simulink model "V.1.3.SystemsmModelling_Modified_Aircorn"  (R2020a)
settings: Solver=ode23t  StartTime=0.0  StopTime=2000  MaxStep=2000.0  RelTol=1e-3
values from neighbouring files (symbols this model uses):
  InitialTemp = 300    [Setup.m]
undefined symbols (not defined in the file or in its folder): commanded_mass_flow, compressor_time_constant, condenser_length, copper_density, environment_temperature, evaporator_length, ground_temperature, pipe_diameter, pipe_thickness, target_temperature, temperature_delta, u_sat
libraries: fl_lib x55, nesl_utility x8, refrigeration_lib x1
(part 3 of 3)

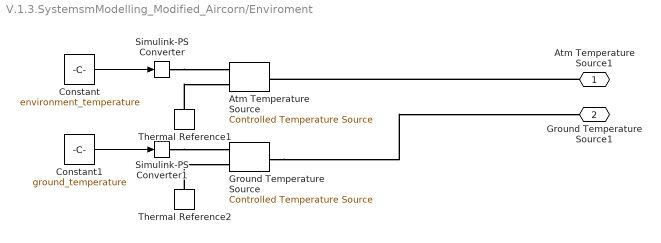
== system V.1.3.SystemsmModelling_Modified_Aircorn/Enviroment ==
  Atm Temperature Source : fl_lib/Thermal/Thermal Sources/Controlled Temperature Source
  Constant : Constant  Value=environment_temperature
  Constant1 : Constant  Value=ground_temperature
  Ground Temperature Source : fl_lib/Thermal/Thermal Sources/Controlled Temperature Source
  Simulink-PS Converter : nesl_utility/Simulink-PS Converter  PhysicalDomain=network_engine_domain  SubClassName=ps_input  LeftPortType=input  RightPortType=output  PseudoPeriodic=off  Frequencies=[]  NoiseDistribution=none  NoiseParameters=[]  Unit=1  AffineConversion=off  FilteringAndDerivatives=provide  SimscapeFilterOrder=1  InputFilterTimeConstant=0.001  UdotUserProvided=0
  Simulink-PS Converter1 : nesl_utility/Simulink-PS Converter  PhysicalDomain=network_engine_domain  SubClassName=ps_input  LeftPortType=input  RightPortType=output  PseudoPeriodic=off  Frequencies=[]  NoiseDistribution=none  NoiseParameters=[]  Unit=1  AffineConversion=off  FilteringAndDerivatives=provide  SimscapeFilterOrder=1  InputFilterTimeConstant=0.001  UdotUserProvided=0
  Thermal Reference1 : fl_lib/Thermal/Thermal Elements/Thermal Reference
  Thermal Reference2 : fl_lib/Thermal/Thermal Elements/Thermal Reference
  Atm Temperature Source1 : PMIOPort  Side=Left
  Ground Temperature Source1 : PMIOPort  Port=2  Side=Left
  wires:
  Constant/1 -> Simulink-PS Converter/1
  Constant1/1 -> Simulink-PS Converter1/1
  connections:
  Thermal Reference2/LConn1 -- Ground Temperature Source/RConn2
  Thermal Reference1/LConn1 -- Atm Temperature Source/RConn2
  Simulink-PS Converter1/RConn1 -- Ground Temperature Source/RConn1
  Ground Temperature Source/LConn1 -- Ground Temperature Source1/RConn1
  Atm Temperature Source1/RConn1 -- Atm Temperature Source/LConn1
  Simulink-PS Converter/RConn1 -- Atm Temperature Source/RConn1

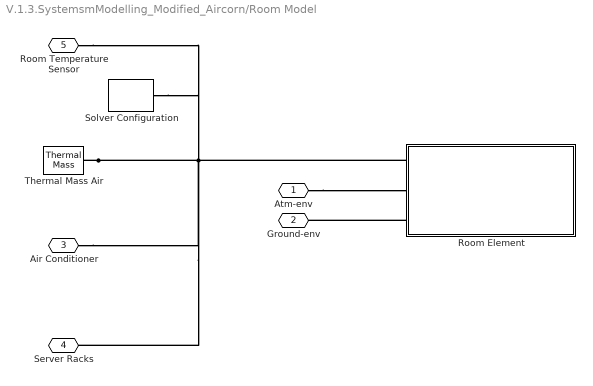
== system V.1.3.SystemsmModelling_Modified_Aircorn/Room Model ==
  "Room Element " : Subsystem
  Solver Configuration : nesl_utility/Solver Configuration  PhysicalDomain=network_engine_domain  SubClassName=solver  LeftPortType=input  RightPortType=generic  Tones=[]  Harmonics=[]  SimulateNoise=off  Profile=off  UseLocalSampling=off  EnableSwitchedLinearOptims=on  FrequencyDomain=off  UseCCode=off  RelTol=0.001  AbsTol=1e-06  MinStep=1e-09  ToWorkspace=off  RevertToSquareIcSolve=off  NumHomotopyIterations=100  PhasorMode=off  PhasorModeNumHarmonics=1  DoDC=off  ResidualTolerance=1e-09  UseLocalSolver=off  LocalSolverChoice=NE_BACKWARD_EULER_ADVANCER  LocalSolverSampleTime=0.001  DoFixedCost=off  MaxNonlinIter=3  MaxModeIter=2  LinearAlgebra=auto  EquationFormulation=NE_TIME_EF  DelaysMemoryBudget=1024  AutomaticFiltering=on  FilteringTimeConstant=0.001  PartitionStorageMethod=AS_NEEDED  PartitionMemoryBudget=1024  PartitionMethod=ROBUST
  Thermal Mass Air : fl_lib/Thermal/Thermal Elements/Thermal Mass  mass=1 kg  sp_heat=1012 J/kg/K  T_specify=off  T_priority=High  T=300 K  T_nominal_specify=off  T_nominal_unit=K  T_nominal_value=1  Q_specify=off  Q_priority=None  Q=0 W  Q_nominal_specify=off  Q_nominal_unit=W  Q_nominal_value=1
  Atm-env : PMIOPort  Side=Left
  Ground-env : PMIOPort  Port=2  Side=Left
  Air Conditioner : PMIOPort  Port=3  Side=Left
  Server Racks : PMIOPort  Port=4  Side=Left
  "Room Temperature Sensor " : PMIOPort  Port=5  Side=Left
  connections:
  Thermal Mass Air/LConn1 -- Server Racks/RConn1 -- Air Conditioner/RConn1 -- "Room Temperature Sensor "/RConn1 -- Solver Configuration/RConn1 -- "Room Element "/LConn1
  Atm-env/RConn1 -- "Room Element "/LConn2
  "Room Element "/LConn3 -- Ground-env/RConn1

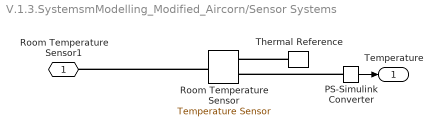
== system V.1.3.SystemsmModelling_Modified_Aircorn/Sensor Systems ==
  PS-Simulink Converter : nesl_utility/PS-Simulink Converter  PhysicalDomain=network_engine_domain  SubClassName=ps_output  LeftPortType=input  RightPortType=output  PseudoPeriodic=off  Frequencies=[]  Unit=inherit  AffineConversion=off
  Room Temperature Sensor : fl_lib/Thermal/Thermal Sensors/Temperature Sensor
  Thermal Reference : fl_lib/Thermal/Thermal Elements/Thermal Reference
  Room Temperature Sensor1 : PMIOPort  Side=Left
  "Temperature " : Outport
  wires:
  PS-Simulink Converter/1 -> "Temperature "/1
  connections:
  PS-Simulink Converter/LConn1 -- Room Temperature Sensor/RConn2
  Thermal Reference/LConn1 -- Room Temperature Sensor/RConn1
  Room Temperature Sensor/LConn1 -- Room Temperature Sensor1/RConn1

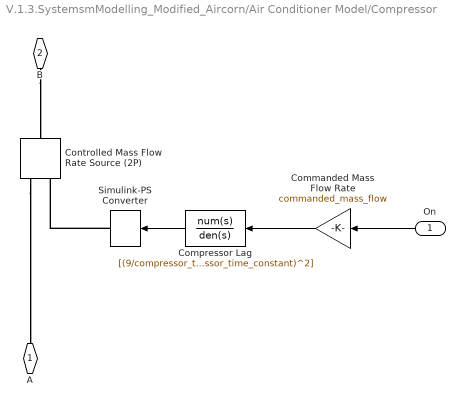
== system V.1.3.SystemsmModelling_Modified_Aircorn/Air Conditioner Model/Compressor ==
  On : Inport
  Commanded Mass Flow Rate : Gain  Gain=commanded_mass_flow
  Compressor Lag : TransferFcn  Numerator=[(9/compressor_time_constant)^2]  Denominator=[1, 2*(9/compressor_time_constant), (9/compressor_time_constant)^2]
  Controlled Mass Flow Rate Source (2P) : fl_lib/Two-Phase Fluid/Sources/Controlled Mass Flow Rate Source (2P)  power_spec=foundation.enum.power_spec.isentropic  area_A=pi*pipe_diameter^2/4 m^2  area_B=pi*pipe_diameter^2/4 m^2
      settings: SourceProductBaseCode=SS  InternalSimscapePortConfiguration="{\"Bottom\":[],\"Left\":[{\"id\":\"A\",\"label\":\"A\",\"type\":\"foundation.two_phase_fluid.two_phase_fluid\"},{\"id\":\"M\",\"label\":\"M\",\"type\":\"input\"}],\"Right\":[{\"id\":\"B\",\"label\":\"B\",\"type\":\"foundation.two_phase_fluid.two_phase_fluid\"}],\"Top\":[]}"
  Simulink-PS Converter : nesl_utility/Simulink-PS Converter  PhysicalDomain=network_engine_domain  SubClassName=ps_input  LeftPortType=input  RightPortType=output  PseudoPeriodic=off  Frequencies=[]  NoiseDistribution=none  NoiseParameters=[]  Unit=kg/s  AffineConversion=off  FilteringAndDerivatives=zero  SimscapeFilterOrder=1  InputFilterTimeConstant=0.001  UdotUserProvided=1
  A : PMIOPort  Side=Left
  B : PMIOPort  Port=2  Side=Right
  wires:
  Compressor Lag/1 -> Simulink-PS Converter/1
  Commanded Mass Flow Rate/1 -> Compressor Lag/1
  On/1 -> Commanded Mass Flow Rate/1
  connections:
  Simulink-PS Converter/RConn1 -- Controlled Mass Flow Rate Source (2P)/LConn2
  Controlled Mass Flow Rate Source (2P)/LConn1 -- A/RConn1
  B/RConn1 -- Controlled Mass Flow Rate Source (2P)/RConn1

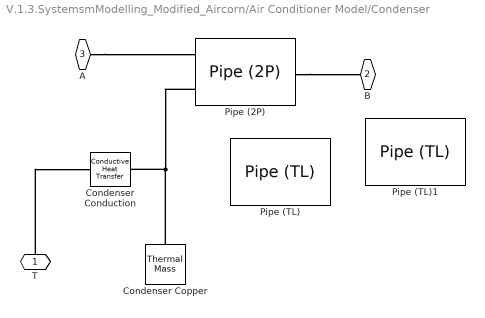
== system V.1.3.SystemsmModelling_Modified_Aircorn/Air Conditioner Model/Condenser ==
  Condenser Conduction : fl_lib/Thermal/Thermal Elements/Conductive Heat Transfer  area=pi*pipe_diameter*condenser_length m^2  thickness=pipe_thickness m  th_cond=copper_conductivity W/(m*K)  T_specify=off  T_priority=High  T=0 K  T_nominal_specify=off  T_nominal_unit=K  T_nominal_value=1  Q_specify=off  Q_priority=High  Q=0 J/s  Q_nominal_specify=off  Q_nominal_unit=W  Q_nominal_value=1
  Condenser Copper : fl_lib/Thermal/Thermal Elements/Thermal Mass  mass=pi*pipe_diameter*condenser_length*pipe_thickness*copper_density kg  sp_heat=copper_specific_heat J/kg/K  T_specify=on  T_priority=High  T=environment_temperature K  T_nominal_specify=off  T_nominal_unit=K  T_nominal_value=1  Q_specify=off  Q_priority=High  Q=0 J/s  Q_nominal_specify=off  Q_nominal_unit=W  Q_nominal_value=1
  Pipe (2P) : fl_lib/Two-Phase Fluid/Elements/Pipe (2P)  length=condenser_length m  area=pi*pipe_diameter^2/4 m^2  Dh=pipe_diameter m  length_add=0.1*condenser_length m  roughness=15e-6 m  Re_lam=2000  Re_tur=4000  shape_factor=64  Nu_lam=5  inertia=simscape.enum.onoff.off  energy_spec=foundation.enum.energy_spec.temperature  p_init=charge_pressure MPa  T_init=-1 K  x_init=0.5  alpha_init=0.5  h_init=1500 kJ/kg  u_init=1500 kJ/kg  mdot_init=0 kg/s  time_constant=0.1 s
      settings: SourceProductBaseCode=SS  InternalSimscapePortConfiguration="{\"Bottom\":[],\"Left\":[{\"id\":\"A\",\"label\":\"A\",\"type\":\"foundation.two_phase_fluid.two_phase_fluid\"},{\"id\":\"H\",\"label\":\"H\",\"type\":\"foundation.thermal.thermal\"}],\"Right\":[{\"id\":\"B\",\"label\":\"B\",\"type\":\"foundation.two_phase_fluid.two_phase_fluid\"}],\"Top\":[]}"
  Pipe (TL) : fl_lib/Thermal Liquid/Elements/Pipe (TL)  length=5 m  area=0.01 m^2  Dh=0.1128 m  length_add=1 m  roughness=15e-6 m  Re_lam=2000  Re_tur=4000  shape_factor=64  Nu_lam=3.66  dynamic_compressibility=simscape.enum.onoff.on  inertia=simscape.enum.onoff.off  p0=0.101325 MPa  T0=293.15 K  mdot0=0 kg/s
      settings: SourceProductBaseCode=SS
  Pipe (TL)1 : fl_lib/Thermal Liquid/Elements/Pipe (TL)  length=5 m  area=0.01 m^2  Dh=0.1128 m  length_add=1 m  roughness=15e-6 m  Re_lam=2000  Re_tur=4000  shape_factor=64  Nu_lam=3.66  dynamic_compressibility=simscape.enum.onoff.on  inertia=simscape.enum.onoff.off  p0=0.101325 MPa  T0=293.15 K  mdot0=0 kg/s
      settings: SourceProductBaseCode=SS
  T : PMIOPort  Side=Left
  B : PMIOPort  Port=2  Side=Left
  A : PMIOPort  Port=3  Side=Right
  connections:
  Condenser Copper/LConn1 -- Pipe (2P)/LConn2 -- Condenser Conduction/LConn1
  T/RConn1 -- Condenser Conduction/RConn1
  A/RConn1 -- Pipe (2P)/LConn1
  Pipe (2P)/RConn1 -- B/RConn1

== system V.1.3.SystemsmModelling_Modified_Aircorn/Air Conditioner Model/Control ==
  Err : Inport
  Relay : Relay  OnSwitchValue=temperature_delta  OffSwitchValue=-temperature_delta
  On : Outport
  wires:
  Err/1 -> Relay/1
  Relay/1 -> On/1

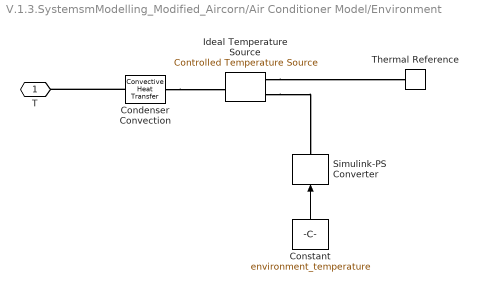
== system V.1.3.SystemsmModelling_Modified_Aircorn/Air Conditioner Model/Environment ==
  Condenser Convection : fl_lib/Thermal/Thermal Elements/Convective Heat Transfer  area=fin_area m^2  heat_tr_coeff=fin_convection_coefficient W/(m^2 * K)  T_specify=off  T_priority=High  T=0 K  T_nominal_specify=off  T_nominal_unit=K  T_nominal_value=1  Q_specify=off  Q_priority=High  Q=0 J/s  Q_nominal_specify=off  Q_nominal_unit=W  Q_nominal_value=1
  Constant : Constant  Value=environment_temperature
  Ideal Temperature Source : fl_lib/Thermal/Thermal Sources/Controlled Temperature Source
  Simulink-PS Converter : nesl_utility/Simulink-PS Converter  PhysicalDomain=network_engine_domain  SubClassName=ps_input  LeftPortType=input  RightPortType=output  PseudoPeriodic=off  Frequencies=[]  NoiseDistribution=none  NoiseParameters=[]  Unit=K  AffineConversion=off  FilteringAndDerivatives=zero  SimscapeFilterOrder=1  InputFilterTimeConstant=0.001  UdotUserProvided=1
  Thermal Reference : fl_lib/Thermal/Thermal Elements/Thermal Reference
  T : PMIOPort  Side=Left
  wires:
  Constant/1 -> Simulink-PS Converter/1
  connections:
  Condenser Convection/RConn1 -- Ideal Temperature Source/LConn1
  Condenser Convection/LConn1 -- T/RConn1
  Ideal Temperature Source/RConn1 -- Simulink-PS Converter/RConn1
  Ideal Temperature Source/RConn2 -- Thermal Reference/LConn1

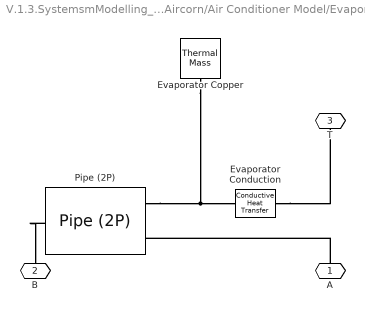
== system V.1.3.SystemsmModelling_Modified_Aircorn/Air Conditioner Model/Evaporator ==
  Evaporator Conduction : fl_lib/Thermal/Thermal Elements/Conductive Heat Transfer  area=pi*pipe_diameter*evaporator_length m^2  thickness=pipe_thickness m  th_cond=copper_conductivity W/(m*K)  T_specify=off  T_priority=High  T=0 K  T_nominal_specify=off  T_nominal_unit=K  T_nominal_value=1  Q_specify=off  Q_priority=High  Q=0 J/s  Q_nominal_specify=off  Q_nominal_unit=W  Q_nominal_value=1
  Evaporator Copper : fl_lib/Thermal/Thermal Elements/Thermal Mass  mass=pi*pipe_diameter*evaporator_length*pipe_thickness*copper_density kg  sp_heat=copper_specific_heat J/kg/K  T_specify=on  T_priority=High  T=target_temperature K  T_nominal_specify=off  T_nominal_unit=K  T_nominal_value=1  Q_specify=off  Q_priority=High  Q=0 J/s  Q_nominal_specify=off  Q_nominal_unit=W  Q_nominal_value=1
  Pipe (2P) : fl_lib/Two-Phase Fluid/Elements/Pipe (2P)  length=evaporator_length m  area=pi*pipe_diameter^2/4 m^2  Dh=pipe_diameter m  length_add=0.1*evaporator_length m  roughness=15e-6 m  Re_lam=2000  Re_tur=4000  shape_factor=64  Nu_lam=5  inertia=simscape.enum.onoff.off  energy_spec=foundation.enum.energy_spec.temperature  p_init=charge_pressure MPa  T_init=-1 K  x_init=0.5  alpha_init=0.5  h_init=1500 kJ/kg  u_init=1500 kJ/kg  mdot_init=0 kg/s  time_constant=0.1 s
      settings: SourceProductBaseCode=SS  InternalSimscapePortConfiguration="{\"Bottom\":[],\"Left\":[{\"id\":\"A\",\"label\":\"A\",\"type\":\"foundation.two_phase_fluid.two_phase_fluid\"},{\"id\":\"H\",\"label\":\"H\",\"type\":\"foundation.thermal.thermal\"}],\"Right\":[{\"id\":\"B\",\"label\":\"B\",\"type\":\"foundation.two_phase_fluid.two_phase_fluid\"}],\"Top\":[]}"
  A : PMIOPort  Side=Left
  B : PMIOPort  Port=2  Side=Right
  T : PMIOPort  Port=3  Side=Right
  connections:
  Evaporator Conduction/RConn1 -- T/RConn1
  Evaporator Copper/LConn1 -- Pipe (2P)/LConn2 -- Evaporator Conduction/LConn1
  A/RConn1 -- Pipe (2P)/LConn1
  Pipe (2P)/RConn1 -- B/RConn1

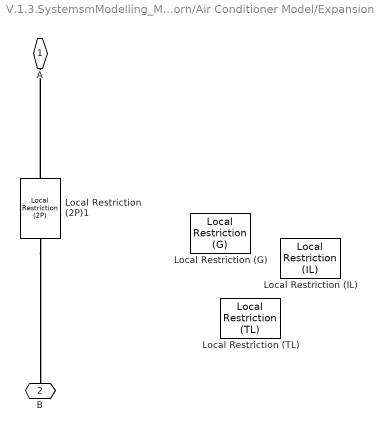
== system V.1.3.SystemsmModelling_Modified_Aircorn/Air Conditioner Model/Expansion Valve ==
  Local Restriction (2P)1 : fl_lib/Two-Phase Fluid/Elements/Local Restriction (2P)  restriction_area=1e-3 m^2  area=pi*pipe_diameter^2/4 m^2  Cd=0.7  B_lam=0.999
      settings: SourceProductBaseCode=SS  InternalSimscapePortConfiguration="{\"Bottom\":[],\"Left\":[{\"id\":\"A\",\"label\":\"A\",\"type\":\"foundation.two_phase_fluid.two_phase_fluid\"}],\"Right\":[{\"id\":\"B\",\"label\":\"B\",\"type\":\"foundation.two_phase_fluid.two_phase_fluid\"}],\"Top\":[]}"
  Local Restriction (G) : fl_lib/Gas/Elements/Local Restriction (G)  restriction_type=foundation.enum.restriction_type.variable  restriction_area=1e-3 m^2  min_area=1e-10 m^2  max_area=0.005 m^2  area=0.01 m^2  Cd=0.64  B_lam=0.999
      settings: SourceProductBaseCode=SS  InternalSimscapePortConfiguration="{\"Bottom\":[],\"Left\":[{\"id\":\"A\",\"label\":\"A\",\"type\":\"foundation.gas.gas\"},{\"id\":\"area_in\",\"label\":\"AR\",\"type\":\"input\"}],\"Right\":[{\"id\":\"B\",\"label\":\"B\",\"type\":\"foundation.gas.gas\"}],\"Top\":[]}"
  Local Restriction (IL) : fl_lib/Isothermal Liquid/Elements/Local Restriction (IL)  restriction_type=foundation.enum.restriction_type.variable  restriction_area=1e-3 m^2  min_area=1e-10 m^2  max_area=0.005 m^2  area=inf m^2  Cd=0.64  Re_c=150  pressure_recovery=simscape.enum.onoff.off
      settings: SourceProductBaseCode=SS  InternalSimscapePortConfiguration="{\"Bottom\":[],\"Left\":[{\"id\":\"A\",\"label\":\"A\",\"type\":\"foundation.isothermal_liquid.isothermal_liquid\"},{\"id\":\"AR\",\"label\":\"AR\",\"type\":\"input\"}],\"Right\":[{\"id\":\"B\",\"label\":\"B\",\"type\":\"foundation.isothermal_liquid.isothermal_liquid\"}],\"Top\":[]}"
  Local Restriction (TL) : fl_lib/Thermal Liquid/Elements/Local Restriction (TL)  restriction_type=foundation.enum.restriction_type.variable  restriction_area=0.001 m^2  min_area=1e-10 m^2  max_area=0.005 m^2  area=0.01 m^2  Cd=0.64  pressure_recovery=simscape.enum.onoff.on  Re_c=12
      settings: SourceProductBaseCode=SS  InternalSimscapePortConfiguration="{\"Bottom\":[],\"Left\":[{\"id\":\"A\",\"label\":\"A\",\"type\":\"foundation.thermal_liquid.thermal_liquid\"},{\"id\":\"area_in\",\"label\":\"AR\",\"type\":\"input\"}],\"Right\":[{\"id\":\"B\",\"label\":\"B\",\"type\":\"foundation.thermal_liquid.thermal_liquid\"}],\"Top\":[]}"
  A : PMIOPort  Side=Left
  B : PMIOPort  Port=2  Side=Right
  connections:
  Local Restriction (2P)1/LConn1 -- A/RConn1
  Local Restriction (2P)1/RConn1 -- B/RConn1

== system V.1.3.SystemsmModelling_Modified_Aircorn/Air Conditioner Model/Plot Properties ==

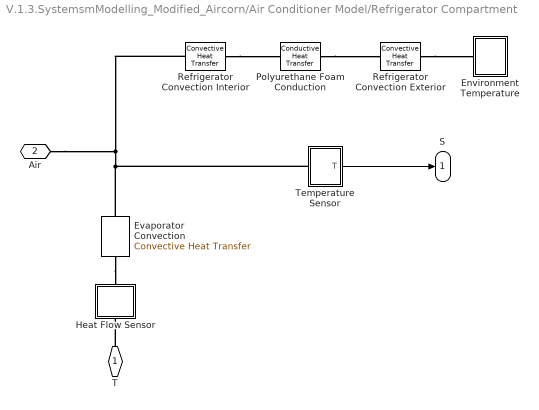
== system V.1.3.SystemsmModelling_Modified_Aircorn/Air Conditioner Model/Refrigerator Compartment ==
  Environment Temperature : Subsystem
  Evaporator Convection : fl_lib/Thermal/Thermal Elements/Convective Heat Transfer  area=interior_surface_area m^2  heat_tr_coeff=natural_convection_coefficient W/(m^2 * K)  T_specify=off  T_priority=High  T=0 K  T_nominal_specify=off  T_nominal_unit=K  T_nominal_value=1  Q_specify=off  Q_priority=High  Q=0 J/s  Q_nominal_specify=off  Q_nominal_unit=W  Q_nominal_value=1
  Heat Flow Sensor : Subsystem
  Polyurethane Foam Conduction : fl_lib/Thermal/Thermal Elements/Conductive Heat Transfer  area=interior_surface_area m^2  thickness=foam_thickness m  th_cond=foam_conductivity W/(m*K)  T_specify=off  T_priority=High  T=0 K  T_nominal_specify=off  T_nominal_unit=K  T_nominal_value=1  Q_specify=off  Q_priority=High  Q=0 J/s  Q_nominal_specify=off  Q_nominal_unit=W  Q_nominal_value=1
  Refrigerator Convection Exterior : fl_lib/Thermal/Thermal Elements/Convective Heat Transfer  area=exterior_surface_area m^2  heat_tr_coeff=natural_convection_coefficient W/(m^2 * K)  T_specify=off  T_priority=High  T=0 K  T_nominal_specify=off  T_nominal_unit=K  T_nominal_value=1  Q_specify=off  Q_priority=High  Q=0 J/s  Q_nominal_specify=off  Q_nominal_unit=W  Q_nominal_value=1
  Refrigerator Convection Interior : fl_lib/Thermal/Thermal Elements/Convective Heat Transfer  area=interior_surface_area m^2  heat_tr_coeff=natural_convection_coefficient W/(m^2 * K)  T_specify=off  T_priority=High  T=0 K  T_nominal_specify=off  T_nominal_unit=K  T_nominal_value=1  Q_specify=off  Q_priority=High  Q=0 J/s  Q_nominal_specify=off  Q_nominal_unit=W  Q_nominal_value=1
  Temperature Sensor : Subsystem
  T : PMIOPort  Side=Left
  Air : PMIOPort  Port=2  Side=Left
  S : Outport
  wires:
  Temperature Sensor/1(T) -> S/1
  connections:
  Evaporator Convection/LConn1 -- Heat Flow Sensor/RConn1
  T/RConn1 -- Heat Flow Sensor/LConn1
  Refrigerator Convection Exterior/RConn1 -- Environment Temperature/LConn1
  Refrigerator Convection Interior/LConn1 -- Evaporator Convection/RConn1 -- Temperature Sensor/LConn1 -- Air/RConn1
  Refrigerator Convection Interior/RConn1 -- Polyurethane Foam Conduction/LConn1
  Polyurethane Foam Conduction/RConn1 -- Refrigerator Convection Exterior/LConn1

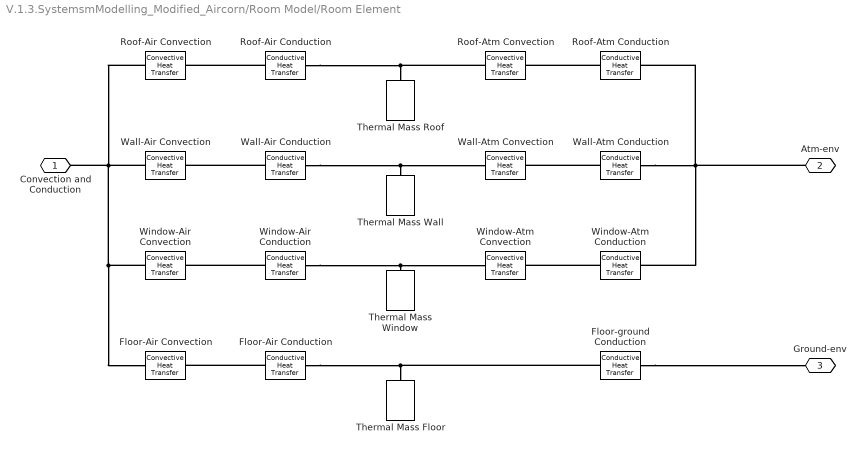
== system V.1.3.SystemsmModelling_Modified_Aircorn/Room Model/Room Element  ==
  " Wall-Air Conduction" : fl_lib/Thermal/Thermal Elements/Conductive Heat Transfer  area=375 m^2  thickness=0.2 m  th_cond=0.15 W/(m*K)  T_specify=off  T_priority=None  T=0 K  T_nominal_specify=off  T_nominal_unit=K  T_nominal_value=1  Q_specify=off  Q_priority=None  Q=0 W  Q_nominal_specify=off  Q_nominal_unit=W  Q_nominal_value=1
  " Wall-Atm Conduction" : fl_lib/Thermal/Thermal Elements/Conductive Heat Transfer  area=375 m^2  thickness=0.2 m  th_cond=0.15 W/(m*K)  T_specify=off  T_priority=None  T=0 K  T_nominal_specify=off  T_nominal_unit=K  T_nominal_value=1  Q_specify=off  Q_priority=None  Q=0 W  Q_nominal_specify=off  Q_nominal_unit=W  Q_nominal_value=1
  " Window-Air Conduction" : fl_lib/Thermal/Thermal Elements/Conductive Heat Transfer  area=25 m^2  thickness=0.2 m  th_cond=0.96 W/(m*K)  T_specify=off  T_priority=None  T=0 K  T_nominal_specify=off  T_nominal_unit=K  T_nominal_value=1  Q_specify=off  Q_priority=None  Q=0 W  Q_nominal_specify=off  Q_nominal_unit=W  Q_nominal_value=1
  " Window-Atm Conduction" : fl_lib/Thermal/Thermal Elements/Conductive Heat Transfer  area=25 m^2  thickness=0.2 m  th_cond=0.96 W/(m*K)  T_specify=off  T_priority=None  T=0 K  T_nominal_specify=off  T_nominal_unit=K  T_nominal_value=1  Q_specify=off  Q_priority=None  Q=0 W  Q_nominal_specify=off  Q_nominal_unit=W  Q_nominal_value=1
  Floor-Air Conduction : fl_lib/Thermal/Thermal Elements/Conductive Heat Transfer  area=25 m^2  thickness=0.2 m  th_cond=0.96 W/(m*K)  T_specify=off  T_priority=None  T=0 K  T_nominal_specify=off  T_nominal_unit=K  T_nominal_value=1  Q_specify=off  Q_priority=None  Q=0 W  Q_nominal_specify=off  Q_nominal_unit=W  Q_nominal_value=1
  Floor-Air Convection : fl_lib/Thermal/Thermal Elements/Convective Heat Transfer  area=20 m^2  heat_tr_coeff=3.3 W/(m^2 * K)  T_specify=off  T_priority=None  T=0 K  T_nominal_specify=off  T_nominal_unit=K  T_nominal_value=1  Q_specify=off  Q_priority=None  Q=0 W  Q_nominal_specify=off  Q_nominal_unit=W  Q_nominal_value=1
  Floor-ground Conduction : fl_lib/Thermal/Thermal Elements/Conductive Heat Transfer  area=25 m^2  thickness=0.2 m  th_cond=0.96 W/(m*K)  T_specify=off  T_priority=None  T=0 K  T_nominal_specify=off  T_nominal_unit=K  T_nominal_value=1  Q_specify=off  Q_priority=None  Q=0 W  Q_nominal_specify=off  Q_nominal_unit=W  Q_nominal_value=1
  Roof-Air Conduction : fl_lib/Thermal/Thermal Elements/Conductive Heat Transfer  area=100 m^2  thickness=0.2 m  th_cond=0.12 W/(m*K)  T_specify=off  T_priority=None  T=0 K  T_nominal_specify=off  T_nominal_unit=K  T_nominal_value=1  Q_specify=off  Q_priority=None  Q=0 W  Q_nominal_specify=off  Q_nominal_unit=W  Q_nominal_value=1
  Roof-Air Convection : fl_lib/Thermal/Thermal Elements/Convective Heat Transfer  area=100 m^2  heat_tr_coeff=20 W/(m^2 * K)  T_specify=off  T_priority=None  T=0 K  T_nominal_specify=off  T_nominal_unit=K  T_nominal_value=1  Q_specify=off  Q_priority=None  Q=0 W  Q_nominal_specify=off  Q_nominal_unit=W  Q_nominal_value=1
  Roof-Atm Conduction : fl_lib/Thermal/Thermal Elements/Conductive Heat Transfer  area=100 m^2  thickness=0.2 m  th_cond=0.12 W/(m*K)  T_specify=off  T_priority=None  T=0 K  T_nominal_specify=off  T_nominal_unit=K  T_nominal_value=1  Q_specify=off  Q_priority=None  Q=0 W  Q_nominal_specify=off  Q_nominal_unit=W  Q_nominal_value=1
  Roof-Atm Convection : fl_lib/Thermal/Thermal Elements/Convective Heat Transfer  area=100 m^2  heat_tr_coeff=20 W/(m^2 * K)  T_specify=off  T_priority=None  T=0 K  T_nominal_specify=off  T_nominal_unit=K  T_nominal_value=1  Q_specify=off  Q_priority=None  Q=0 W  Q_nominal_specify=off  Q_nominal_unit=W  Q_nominal_value=1
  Thermal Mass Floor : fl_lib/Thermal/Thermal Elements/Thermal Mass  mass=48 kg  sp_heat=840.7 J/kg/K  T_specify=on  T_priority=High  T=InitialTemp K  T_nominal_specify=off  T_nominal_unit=K  T_nominal_value=1  Q_specify=off  Q_priority=None  Q=0 W  Q_nominal_specify=off  Q_nominal_unit=W  Q_nominal_value=1
  Thermal Mass Roof : fl_lib/Thermal/Thermal Elements/Thermal Mass  mass=48 kg  sp_heat=853.7 J/kg/K  T_specify=on  T_priority=High  T=InitialTemp K  T_nominal_specify=off  T_nominal_unit=K  T_nominal_value=1  Q_specify=off  Q_priority=None  Q=0 W  Q_nominal_specify=off  Q_nominal_unit=W  Q_nominal_value=1
  Thermal Mass Wall : fl_lib/Thermal/Thermal Elements/Thermal Mass  mass=180 kg  sp_heat=868.2 J/kg/K  T_specify=on  T_priority=High  T=InitialTemp K  T_nominal_specify=off  T_nominal_unit=K  T_nominal_value=1  Q_specify=off  Q_priority=None  Q=0 W  Q_nominal_specify=off  Q_nominal_unit=W  Q_nominal_value=1
  Thermal Mass Window : fl_lib/Thermal/Thermal Elements/Thermal Mass  mass=11 kg  sp_heat=840 J/kg/K  T_specify=on  T_priority=High  T=InitialTemp K  T_nominal_specify=off  T_nominal_unit=K  T_nominal_value=1  Q_specify=off  Q_priority=None  Q=0 W  Q_nominal_specify=off  Q_nominal_unit=W  Q_nominal_value=1
  Wall-Air Convection : fl_lib/Thermal/Thermal Elements/Convective Heat Transfer  area=375 m^2  heat_tr_coeff=20 W/(m^2 * K)  T_specify=off  T_priority=None  T=0 K  T_nominal_specify=off  T_nominal_unit=K  T_nominal_value=1  Q_specify=off  Q_priority=None  Q=0 W  Q_nominal_specify=off  Q_nominal_unit=W  Q_nominal_value=1
  Wall-Atm Convection : fl_lib/Thermal/Thermal Elements/Convective Heat Transfer  area=375 m^2  heat_tr_coeff=20 W/(m^2 * K)  T_specify=off  T_priority=None  T=0 K  T_nominal_specify=off  T_nominal_unit=K  T_nominal_value=1  Q_specify=off  Q_priority=None  Q=0 W  Q_nominal_specify=off  Q_nominal_unit=W  Q_nominal_value=1
  Window-Air Convection : fl_lib/Thermal/Thermal Elements/Convective Heat Transfer  area=25 m^2  heat_tr_coeff=3.3 W/(m^2 * K)  T_specify=off  T_priority=None  T=0 K  T_nominal_specify=off  T_nominal_unit=K  T_nominal_value=1  Q_specify=off  Q_priority=None  Q=0 W  Q_nominal_specify=off  Q_nominal_unit=W  Q_nominal_value=1
  Window-Atm Convection : fl_lib/Thermal/Thermal Elements/Convective Heat Transfer  area=25 m^2  heat_tr_coeff=3.3 W/(m^2 * K)  T_specify=off  T_priority=None  T=0 K  T_nominal_specify=off  T_nominal_unit=K  T_nominal_value=1  Q_specify=off  Q_priority=None  Q=0 W  Q_nominal_specify=off  Q_nominal_unit=W  Q_nominal_value=1
  Convection and Conduction : PMIOPort  Side=Left
  Atm-env : PMIOPort  Port=2  Side=Left
  Ground-env : PMIOPort  Port=3  Side=Left
  connections:
  " Window-Atm Conduction"/RConn1 -- Window-Atm Convection/LConn1
  Floor-ground Conduction/LConn1 -- Ground-env/RConn1
  Roof-Air Conduction/RConn1 -- Roof-Air Convection/LConn1
  Floor-Air Conduction/LConn1 -- Floor-ground Conduction/RConn1 -- Thermal Mass Floor/LConn1
  " Wall-Atm Conduction"/LConn1 -- Atm-env/RConn1 -- Roof-Atm Conduction/LConn1 -- " Window-Atm Conduction"/LConn1
  Roof-Air Convection/RConn1 -- Convection and Conduction/RConn1 -- Window-Air Convection/RConn1 -- Floor-Air Convection/RConn1 -- Wall-Air Convection/RConn1
  Roof-Atm Convection/RConn1 -- Roof-Air Conduction/LConn1 -- Thermal Mass Roof/LConn1
  Roof-Atm Conduction/RConn1 -- Roof-Atm Convection/LConn1
  " Wall-Air Conduction"/LConn1 -- Wall-Atm Convection/RConn1 -- Thermal Mass Wall/LConn1
  " Window-Air Conduction"/LConn1 -- Window-Atm Convection/RConn1 -- Thermal Mass Window/LConn1
  " Wall-Atm Conduction"/RConn1 -- Wall-Atm Convection/LConn1
  " Wall-Air Conduction"/RConn1 -- Wall-Air Convection/LConn1
  " Window-Air Conduction"/RConn1 -- Window-Air Convection/LConn1
  Floor-Air Conduction/RConn1 -- Floor-Air Convection/LConn1

== system V.1.3.SystemsmModelling_Modified_Aircorn/Air Conditioner Model/Refrigerator Compartment/Environment Temperature ==
  Constant : Constant  Value=environment_temperature
  Ideal Temperature Source : fl_lib/Thermal/Thermal Sources/Controlled Temperature Source
  Simulink-PS Converter : nesl_utility/Simulink-PS Converter  PhysicalDomain=network_engine_domain  SubClassName=ps_input  LeftPortType=input  RightPortType=output  PseudoPeriodic=off  Frequencies=[]  NoiseDistribution=none  NoiseParameters=[]  Unit=K  AffineConversion=off  FilteringAndDerivatives=zero  SimscapeFilterOrder=1  InputFilterTimeConstant=0.001  UdotUserProvided=1
  Thermal Reference : fl_lib/Thermal/Thermal Elements/Thermal Reference
  T : PMIOPort  Side=Left
  wires:
  Constant/1 -> Simulink-PS Converter/1
  connections:
  Ideal Temperature Source/RConn2 -- Thermal Reference/LConn1
  Ideal Temperature Source/RConn1 -- Simulink-PS Converter/RConn1
  Ideal Temperature Source/LConn1 -- T/RConn1

== system V.1.3.SystemsmModelling_Modified_Aircorn/Air Conditioner Model/Refrigerator Compartment/Heat Flow Sensor ==
  Ideal Heat Flow Sensor : fl_lib/Thermal/Thermal Sensors/Heat Flow Rate Sensor
      settings: SourceProductBaseCode=SS
  B : PMIOPort  Side=Right
  A : PMIOPort  Port=2  Side=Left
  connections:
  Ideal Heat Flow Sensor/RConn2 -- B/RConn1
  Ideal Heat Flow Sensor/LConn1 -- A/RConn1

== system V.1.3.SystemsmModelling_Modified_Aircorn/Air Conditioner Model/Refrigerator Compartment/Temperature Sensor ==
  Ideal Temperature Sensor : fl_lib/Thermal/Thermal Sensors/Temperature Sensor
  PS-Simulink Converter : nesl_utility/PS-Simulink Converter  PhysicalDomain=network_engine_domain  SubClassName=ps_output  LeftPortType=input  RightPortType=output  PseudoPeriodic=off  Frequencies=[]  Unit=K  AffineConversion=off
  Thermal Reference : fl_lib/Thermal/Thermal Elements/Thermal Reference
  A : PMIOPort  Side=Left
  T : Outport
  wires:
  PS-Simulink Converter/1 -> T/1
  connections:
  Ideal Temperature Sensor/LConn1 -- A/RConn1
  Thermal Reference/LConn1 -- Ideal Temperature Sensor/RConn1
  PS-Simulink Converter/LConn1 -- Ideal Temperature Sensor/RConn2
